simulink model "correlation_simu"  (R2015a)
settings: Solver=ode45  StartTime=0.0  StopTime=180  RelTol=1e-3
undefined symbols (not defined in the file or in its folder): currentCFG_correlation_simu_UB, fdesignblkfcn, gcbh, UB
libraries: dspvision x3, dspstat3 x1, dspsnks4 x1, gUSBamplib x1
settings Model: Creator=macfa  LastModifiedBy=BCMI

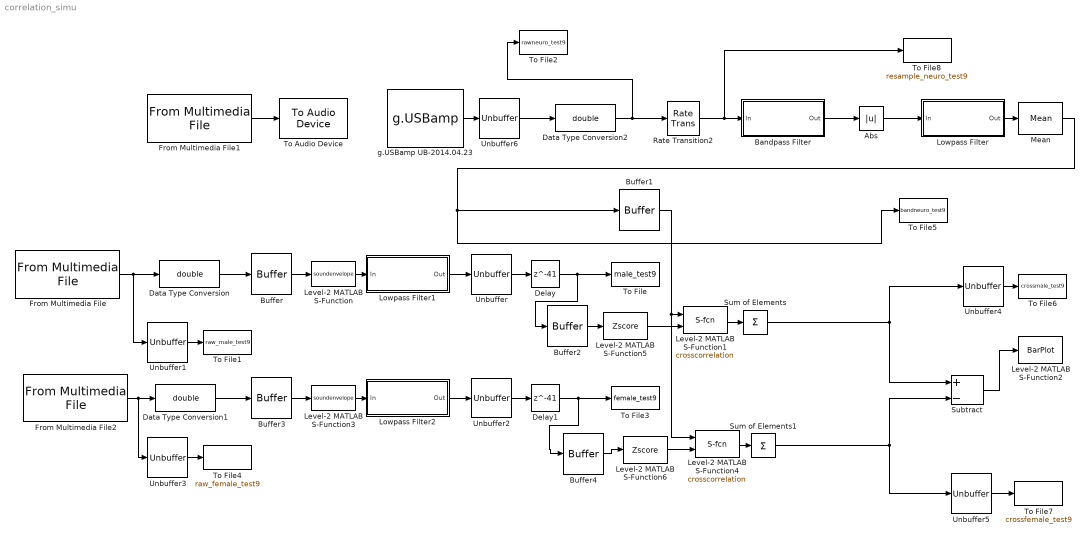
== system correlation_simu ==
  Abs : Abs
  Bandpass Filter : Subsystem  DialogController=fdesignblkfcn  InitFcn=fdesignblkfcn(gcbh, {'InitFcn'});  mask(Bandpass Filter){}
      mask help: Design a bandpass filter
      settings: CopyFcn=fdesignblkfcn(gcbh, {'CopyFcn'});
      mask Help: helpview(mapfilelocation('dsp'), 'dspbandpassfilter');
      mask Display: disp('Bandpass');
  Buffer : Buffer  N=250  TreatMby1Signals=One channel
  Buffer1 : Buffer  N=640  V=640-32  TreatMby1Signals=One channel
  Buffer2 : Buffer  N=640  V=640-32  TreatMby1Signals=One channel
  Buffer3 : Buffer  N=250  TreatMby1Signals=One channel
  Buffer4 : Buffer  N=640  V=640-32  TreatMby1Signals=One channel
  Data Type Conversion : DataTypeConversion  OutDataTypeStr=double
  Data Type Conversion1 : DataTypeConversion  OutDataTypeStr=double
  Data Type Conversion2 : DataTypeConversion  OutDataTypeStr=double
  Delay : Delay  DelayLength=41  InitialCondition=0
  Delay1 : Delay  DelayLength=41  InitialCondition=0
  From Multimedia File : dspvision/From Multimedia File  inputFilename=C:\Users\BCMI\Desktop\fan\MaleOne.wav  loop=on  numPlays=inf  outputStreams=Audio only  videoDataType=single  audioDataType=double  inheritSampleTime=on  userDefinedSampleTime=1/30  noAudioOutput=off  isIntensityVideo=off  fourcc=RGB  colorVideoFormat=Separate color signals  outputEOF=off  dataOrg=Column-major  audioFrameSize=1  computeAudioFrameSize=off  outSamplingMode=Sample based
  From Multimedia File1 : dspvision/From Multimedia File  inputFilename=C:\Users\BCMI\Desktop\fan\MaleOneFemaleTwo.wav  loop=on  numPlays=inf  outputStreams=Audio only  videoDataType=single  audioDataType=double  inheritSampleTime=on  userDefinedSampleTime=1/30  noAudioOutput=off  isIntensityVideo=off  fourcc=RGB  colorVideoFormat=Separate color signals  outputEOF=off  dataOrg=Column-major  audioFrameSize=1  computeAudioFrameSize=off  outSamplingMode=Sample based
  From Multimedia File2 : dspvision/From Multimedia File  inputFilename=C:\Users\BCMI\Desktop\fan\FemaleTwo.wav  loop=on  numPlays=inf  outputStreams=Audio only  videoDataType=single  audioDataType=double  inheritSampleTime=on  userDefinedSampleTime=1/30  noAudioOutput=off  isIntensityVideo=off  fourcc=RGB  colorVideoFormat=Separate color signals  outputEOF=off  dataOrg=Column-major  audioFrameSize=1  computeAudioFrameSize=off  outSamplingMode=Sample based
  Level-2 MATLAB S-Function : M-S-Function  FunctionName=soundenvelope
  Level-2 MATLAB S-Function1 : M-S-Function  FunctionName=crosscorrelation
  Level-2 MATLAB S-Function2 : M-S-Function  FunctionName=BarPlot
  Level-2 MATLAB S-Function3 : M-S-Function  FunctionName=soundenvelope
  Level-2 MATLAB S-Function4 : M-S-Function  FunctionName=crosscorrelation
  Level-2 MATLAB S-Function5 : M-S-Function  FunctionName=Zscore
  Level-2 MATLAB S-Function6 : M-S-Function  FunctionName=Zscore
  Lowpass Filter : Subsystem  DialogController=fdesignblkfcn  InitFcn=fdesignblkfcn(gcbh, {'InitFcn'});  mask(Lowpass Filter){}
      mask help: Design a lowpass filter
      settings: CopyFcn=fdesignblkfcn(gcbh, {'CopyFcn'});
      mask Help: helpview(mapfilelocation('dsp'), 'dsplowpassfilter');
      mask Display: disp('Lowpass')
  Lowpass Filter1 : Subsystem  DialogController=fdesignblkfcn  InitFcn=fdesignblkfcn(gcbh, {'InitFcn'});  mask(Lowpass Filter){}
      mask help: Design a lowpass filter
      settings: CopyFcn=fdesignblkfcn(gcbh, {'CopyFcn'});
      mask Help: helpview(mapfilelocation('dsp'), 'dsplowpassfilter');
      mask Display: disp('Lowpass')
  Lowpass Filter2 : Subsystem  DialogController=fdesignblkfcn  InitFcn=fdesignblkfcn(gcbh, {'InitFcn'});  mask(Lowpass Filter){}
      mask help: Design a lowpass filter
      settings: CopyFcn=fdesignblkfcn(gcbh, {'CopyFcn'});
      mask Help: helpview(mapfilelocation('dsp'), 'dsplowpassfilter');
      mask Display: disp('Lowpass')
  Mean : dspstat3/Mean  run=off  reset_popup=None  InputProcessing=Columns as channels (frame based)  directionMode=Each row  dimension=1  treatSBRowAsCol=off  roiEnable=off  roiType=Rectangles  roiPortion=Entire ROI  roiOutput=Individual statistics for each ROI  roiFlag=off  outputDataTypeStr=Inherit: Same as accumulator  outputLastDataTypeStr=Inherit: Same as accumulator  outputMin=[]  outputMax=[]  roundingMode=Floor  overflowMode=off
  Rate Transition2 : RateTransition  OutPortSampleTimeOpt=Multiple of input port sample time  OutPortSampleTimeMultiple=4
  Subtract : Sum  Inputs=+-
  Sum of Elements : Sum  Inputs=+
  Sum of Elements1 : Sum  Inputs=+
  To Audio Device : dspsnks4/To Audio Device  deviceName=Default  inheritSampleRate=on  sampleRate=44100  deviceDatatype=Determine from input data type  autoBufferSize=on  bufferSize=4096  queueDuration=1.0  defaultOutputChannelMapping=on  outputChannelMapping=1:2  outputNumUnderrunSamples=off
  To File : ToFile  Filename=male_test9  MatrixName=male_test9
  To File1 : ToFile  Filename=raw_male_test9  MatrixName=raw_male_test9
  To File2 : ToFile  Filename=rawneuro_test9  MatrixName=rawneuro_test9
  To File3 : ToFile  Filename=female_test9  MatrixName=female_test9
  To File4 : ToFile  Filename=raw_female_test9  MatrixName=raw_female_test9
  To File5 : ToFile  Filename=bandneuro_test9  MatrixName=bandneuro_test9
  To File6 : ToFile  Filename=crossmale_test9  MatrixName=crossmale_test9
  To File7 : ToFile  Filename=crossfemale_test9  MatrixName=crossfemale_test9
  To File8 : ToFile  Filename=resample_neuro_test9  MatrixName=resample_neuro_test9
  Unbuffer{,1..6} (7 alike) : Unbuffer  SampleBasedProcessing=Same as frame based
  g.USBamp UB-2014.04.23 : gUSBamplib/g.USBamp  cfg=currentCFG_correlation_simu_UB-2014.04.23.cfg  snr=UB-2014.04.23
  wires:
  From Multimedia File/1 -> Data Type Conversion/1, Unbuffer1/1
  Data Type Conversion/1 -> Buffer/1
  Buffer/1 -> Level-2 MATLAB S-Function/1
  Level-2 MATLAB S-Function/1 -> Lowpass Filter1/1(In)
  Unbuffer1/1 -> To File1/1
  From Multimedia File1/1 -> To Audio Device/1
  Buffer2/1 -> Level-2 MATLAB S-Function5/1
  From Multimedia File2/1 -> Data Type Conversion1/1, Unbuffer3/1
  Data Type Conversion1/1 -> Buffer3/1
  Buffer3/1 -> Level-2 MATLAB S-Function3/1
  Level-2 MATLAB S-Function3/1 -> Lowpass Filter2/1(In)
  Unbuffer3/1 -> To File4/1
  Buffer4/1 -> Level-2 MATLAB S-Function6/1
  Unbuffer/1 -> Delay/1
  Unbuffer2/1 -> Delay1/1
  Level-2 MATLAB S-Function1/1 -> Sum of Elements/1
  Level-2 MATLAB S-Function4/1 -> Sum of Elements1/1
  Bandpass Filter/1(Out) -> Abs/1
  Unbuffer6/1 -> Data Type Conversion2/1
  g.USBamp UB-2014.04.23/1 -> Unbuffer6/1
  Data Type Conversion2/1 -> Rate Transition2/1, To File2/1
  Subtract/1 -> Level-2 MATLAB S-Function2/1
  Unbuffer4/1 -> To File6/1
  Unbuffer5/1 -> To File7/1
  Delay1/1 -> To File3/1, Buffer4/1
  Buffer1/1 -> Level-2 MATLAB S-Function1/1, Level-2 MATLAB S-Function4/1
  Level-2 MATLAB S-Function5/1 -> Level-2 MATLAB S-Function1/2
  Level-2 MATLAB S-Function6/1 -> Level-2 MATLAB S-Function4/2
  Sum of Elements1/1 -> Unbuffer5/1, Subtract/2
  Sum of Elements/1 -> Subtract/1, Unbuffer4/1
  Mean/1 -> Buffer1/1, To File5/1
  Lowpass Filter2/1(Out) -> Unbuffer2/1
  Rate Transition2/1 -> Bandpass Filter/1(In), To File8/1
  Lowpass Filter/1(Out) -> Mean/1
  Abs/1 -> Lowpass Filter/1(In)
  Delay/1 -> To File/1, Buffer2/1
  Lowpass Filter1/1(Out) -> Unbuffer/1

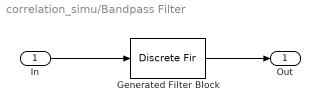
== system correlation_simu/Bandpass Filter ==
  In : Inport
  Generated Filter Block : DiscreteFir  Tag=BlockMethodSubSystem  Coefficients=[7.8110784413432828e-19 0.00057089879376625999 0.00074200256294671319 0.00019878447527332983 -0.0010026233800061598 -0.0022660294618581933 -0.0026799853040919328 -0.0017229844340831977 3.3588243653855798e-18 0.00076454186327833205 -0.0011375888890192735 -0.0057526641048430312 -0.010723729765597791 -0.012545647343105138 -0.0093803901068327672 -0.0033496971516950537 0 -0.0044880349064490019 -0.016868087418978387 -0.03038319223102463 -0.035161558934288503 -0.025720943533778101 -0.0069999521896023558 0.0065486419276123082 -3.0076789781602083e-18 -0.029883629751211026 -0.068008457499660169 -0.086154268007906543 -0.058884391634919667 0.018871554066036803 0.12417621784983256 0.2147863024883413 0.25047248995611254 0.2147863024883413 0.12417621784983256 0.018871554066036803 -0.058884391634919667 -0.086154268007906543 -0.068008457499660169 -0.029883629751211026 -3.0076789781602083e-18 0.0065486419276123082 -0.0069999521896023558 -0.025720943533778101 -0.035161558934288503 -0.03038319223102463 -0.016868087418978387 -0.0044880349064490019 0 -0.0033496971516950537 -0.0093803901068327672 -0.012545647343105138 -0.010723729765597791 -0.0057526641048430312 -0.0011375888890192735 0.00076454186327833205 3.3588243653855798e-18 -0.0017229844340831977 -0.0026799853040919328 -0.0022660294618581933 -0.0010026233800061598 0.00019878447527332983 0.00074200256294671319 0.00057089879376625999 7.8110784413432828e-19]  InputProcessing=Columns as channels (frame based)
  Out : Outport
  wires:
  In/1 -> Generated Filter Block/1
  Generated Filter Block/1 -> Out/1

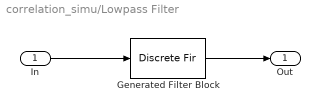
== system correlation_simu/Lowpass Filter ==
  In : Inport
  Generated Filter Block : DiscreteFir  Tag=BlockMethodSubSystem  Coefficients=[-1.9414389490463393e-19 -0.00016404693134369975 -0.00035930547085878016 -0.00060624307855552549 -0.00092092848006727294 -0.00131145669831573 -0.0017747269799691908 -0.002293894851097628 -0.002836783195743423 -0.0033554762712476875 -0.0037872388394997267 -0.0040568057229090774 -0.0040799820490465604 -0.0037683890271385891 -0.0030350923590893282 -0.0018007680299143138 1.3104712906062789e-18 0.0024127284977339303 0.0054577904175328804 0.0091263276482708103 0.013377671053275813 0.018138530083584532 0.023304104903800641 0.028741150291990199 0.034292891037533697 0.039785562227023986 0.04503623367130026 0.049861484049199142 0.054086424044589326 0.057553533888347851 0.060130782091652415 0.061718529102897532 0.062254789952127167 0.061718529102897532 0.060130782091652415 0.057553533888347851 0.054086424044589326 0.049861484049199142 0.04503623367130026 0.039785562227023986 0.034292891037533697 0.028741150291990199 0.023304104903800641 0.018138530083584532 0.013377671053275813 0.0091263276482708103 0.0054577904175328804 0.0024127284977339303 1.3104712906062789e-18 -0.0018007680299143138 -0.0030350923590893282 -0.0037683890271385891 -0.0040799820490465604 -0.0040568057229090774 -0.0037872388394997267 -0.0033554762712476875 -0.002836783195743423 -0.002293894851097628 -0.0017747269799691908 -0.00131145669831573 -0.00092092848006727294 -0.00060624307855552549 -0.00035930547085878016 -0.00016404693134369975 -1.9414389490463393e-19]  InputProcessing=Columns as channels (frame based)
  Out : Outport
  wires:
  In/1 -> Generated Filter Block/1
  Generated Filter Block/1 -> Out/1

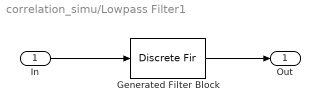
== system correlation_simu/Lowpass Filter1 ==
  In : Inport
  Generated Filter Block : DiscreteFir  Tag=BlockMethodSubSystem  Coefficients=[-1.9414389490463393e-19 -0.00016404693134369975 -0.00035930547085878016 -0.00060624307855552549 -0.00092092848006727294 -0.00131145669831573 -0.0017747269799691908 -0.002293894851097628 -0.002836783195743423 -0.0033554762712476875 -0.0037872388394997267 -0.0040568057229090774 -0.0040799820490465604 -0.0037683890271385891 -0.0030350923590893282 -0.0018007680299143138 1.3104712906062789e-18 0.0024127284977339303 0.0054577904175328804 0.0091263276482708103 0.013377671053275813 0.018138530083584532 0.023304104903800641 0.028741150291990199 0.034292891037533697 0.039785562227023986 0.04503623367130026 0.049861484049199142 0.054086424044589326 0.057553533888347851 0.060130782091652415 0.061718529102897532 0.062254789952127167 0.061718529102897532 0.060130782091652415 0.057553533888347851 0.054086424044589326 0.049861484049199142 0.04503623367130026 0.039785562227023986 0.034292891037533697 0.028741150291990199 0.023304104903800641 0.018138530083584532 0.013377671053275813 0.0091263276482708103 0.0054577904175328804 0.0024127284977339303 1.3104712906062789e-18 -0.0018007680299143138 -0.0030350923590893282 -0.0037683890271385891 -0.0040799820490465604 -0.0040568057229090774 -0.0037872388394997267 -0.0033554762712476875 -0.002836783195743423 -0.002293894851097628 -0.0017747269799691908 -0.00131145669831573 -0.00092092848006727294 -0.00060624307855552549 -0.00035930547085878016 -0.00016404693134369975 -1.9414389490463393e-19]  InputProcessing=Columns as channels (frame based)
  Out : Outport
  wires:
  In/1 -> Generated Filter Block/1
  Generated Filter Block/1 -> Out/1

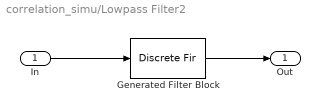
== system correlation_simu/Lowpass Filter2 ==
  In : Inport
  Generated Filter Block : DiscreteFir  Tag=BlockMethodSubSystem  Coefficients=[-1.9414389490463393e-19 -0.00016404693134369975 -0.00035930547085878016 -0.00060624307855552549 -0.00092092848006727294 -0.00131145669831573 -0.0017747269799691908 -0.002293894851097628 -0.002836783195743423 -0.0033554762712476875 -0.0037872388394997267 -0.0040568057229090774 -0.0040799820490465604 -0.0037683890271385891 -0.0030350923590893282 -0.0018007680299143138 1.3104712906062789e-18 0.0024127284977339303 0.0054577904175328804 0.0091263276482708103 0.013377671053275813 0.018138530083584532 0.023304104903800641 0.028741150291990199 0.034292891037533697 0.039785562227023986 0.04503623367130026 0.049861484049199142 0.054086424044589326 0.057553533888347851 0.060130782091652415 0.061718529102897532 0.062254789952127167 0.061718529102897532 0.060130782091652415 0.057553533888347851 0.054086424044589326 0.049861484049199142 0.04503623367130026 0.039785562227023986 0.034292891037533697 0.028741150291990199 0.023304104903800641 0.018138530083584532 0.013377671053275813 0.0091263276482708103 0.0054577904175328804 0.0024127284977339303 1.3104712906062789e-18 -0.0018007680299143138 -0.0030350923590893282 -0.0037683890271385891 -0.0040799820490465604 -0.0040568057229090774 -0.0037872388394997267 -0.0033554762712476875 -0.002836783195743423 -0.002293894851097628 -0.0017747269799691908 -0.00131145669831573 -0.00092092848006727294 -0.00060624307855552549 -0.00035930547085878016 -0.00016404693134369975 -1.9414389490463393e-19]  InputProcessing=Columns as channels (frame based)
  Out : Outport
  wires:
  In/1 -> Generated Filter Block/1
  Generated Filter Block/1 -> Out/1
